simulink model "compansated_design_motor_position"  (R2017b)
settings: Solver=FixedStepAuto  StartTime=0.0  StopTime=inf  FixedStep=0.05  RelTol=1e-3  EnableMultiTasking=on
values from neighbouring files (symbols this model uses):
  rp = 2*pi/(64*gr)    (= 0.00327249234749)    [CL_Constants_PID.m]
libraries: arduinolib x2, THLlib x2
settings Model: ExtModeTrigDuration=2  Creator=sysad  LastModifiedBy=sysad
settings OptimizationCC: PassReuseOutputArgsThreshold=0  MaxStackSize=64
settings DebuggingCC: ParameterTunabilityLossMsg=error
settings HardwareCC: ProdBitPerInt=16  ProdBitPerPointer=16  ProdBitPerSizeT=16  ProdBitPerPtrDiffT=16  ProdLargestAtomicFloat=None  ProdWordSize=8  ProdHWDeviceType=Atmel->AVR  UseEmbeddedCoderFeatures=off
settings SFSimCC: MATLABDynamicMemAlloc=off
settings RTWCC: SystemTargetFile=ert.tlc  HardwareBoard=Arduino Uno  TLCOptions=-aInlineSetEventsForThisBaseRateFcn=TLC_FALSE -aSuppressMultiTaskScheduler=TLC_FALSE -aRateBasedStepFcn=1  TemplateMakefile=ert_default_tmf  GenerateReport=on  Toolchain=Arduino AVR  BuildConfiguration=Faster Runs  LaunchReport=on
settings CodeAppCC: ForceParamTrailComments=on  OperatorAnnotations=on
settings ERTTargetCC: ERTCustomFileBanners=off  SupportContinuousTime=on  SupportNonInlinedSFcns=on  RemoveResetFunc=off  SupportVariableSizeSignals=on  ModelStepFunctionPrototypeControlCompliant=off

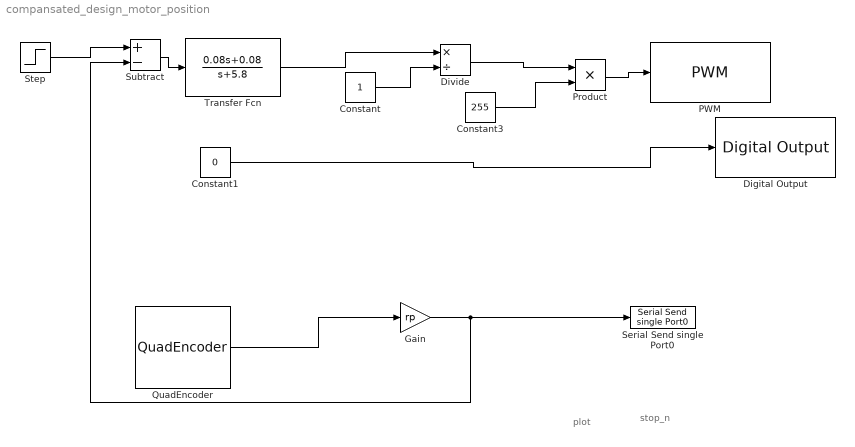
== system compansated_design_motor_position ==
  note: stop_n
  note: plot
  Constant : Constant
  Constant1 : Constant  Value=0
  Constant3 : Constant  Value=255
  Digital Output : arduinolib/Digital Output  pinNumber=4  blockPlatform=arduino
  Divide : Product  Inputs=*/
  Gain : Gain  Gain=rp
  PWM : arduinolib/PWM  pinNumber=5  blockPlatform=arduino
  Product : Product
  QuadEncoder : THLlib/QuadEncoder
      settings: SourceProductName=Take Home Labs Arduino Support Package
  Serial Send single Port0 : THLlib/Serial Send single Port0
      settings: SourceProductName=Take Home Labs Arduino Support Package
  Step : Step  SampleTime=0
  Subtract : Sum  Inputs=+-
  Transfer Fcn : TransferFcn  Numerator=[0.08 0.08]  Denominator=[1 5.8]
  wires:
  Constant/1 -> Divide/2
  Divide/1 -> Product/1
  Constant1/1 -> Digital Output/1
  Product/1 -> PWM/1
  QuadEncoder/1 -> Gain/1
  Constant3/1 -> Product/2
  Gain/1 -> Subtract/2, Serial Send single Port0/1
  Step/1 -> Subtract/1
  Transfer Fcn/1 -> Divide/1
  Subtract/1 -> Transfer Fcn/1
